simulink model "k1vissr2p"  (Simulink 8.6)
settings: Solver=ode45  StartTime=0.0  StopTime=10.0  RelTol=1e-3
libraries: cdsIPCx x11, cdsCDI64 x3, cdsCDO64 x3, TYPEB_MASTER x3, dac x2, cdsAdcx0 x1, cdsParameters x1
settings Model: Creator=controls  LastModifiedBy=controls
settings DataIOCC: SignalLoggingSaveFormat=Dataset
settings OptimizationCC: ExpressionDepthLimit=128
settings DebuggingCC: UnderspecifiedInitializationDetection=Simplified  MergeDetectMultiDrivingBlocksExec=error  SolverPrmCheckMsg=none  FcnCallInpInsideContextMsg=EnableAllAsError  StateNameClashWarn=none
settings GRTTargetCC: CombineOutputUpdateFcns=on  GRTInterface=off

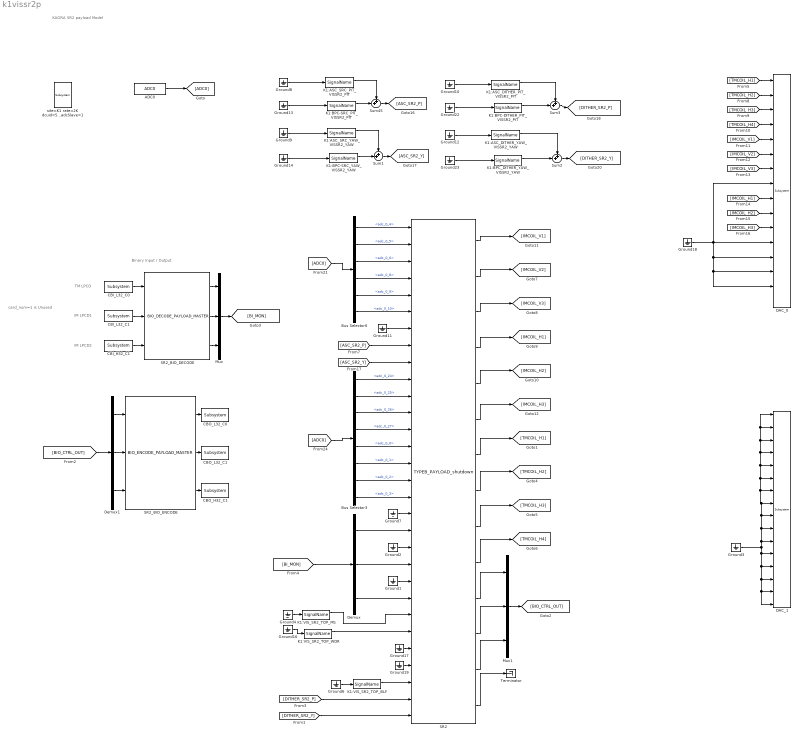
== system k1vissr2p ==
  note: KAGRA SR2 payload Model
  note: TM LPCD
  note: Binary Input / Output
  note: card_num=1 is Unused
  note: IM LPCD1
  note: IM LPCD2
  ADC0 : cdsAdcx0/ADC0  Tag=cdsAdc  Description=|
      | type-GSC_16AI64SSA
      | card_num=0
      settings: AttributesFormatString=%<Description>\n%<Tag>
  Bus Selector3 : BusSelector  Description=ADC Selector  OutputSignals=adc_0_24,adc_0_25,adc_0_26,adc_0_27,adc_0_0,adc_0_1,adc_0_2,adc_0_3
      settings: AttributesFormatString=%<Description>
  Bus Selector6 : BusSelector  Description=ADC Selector  OutputSignals=adc_0_4,adc_0_5,adc_0_6,adc_0_8,adc_0_9,adc_0_10
      settings: AttributesFormatString=%<Description>
  CBI_H32_C1 : cdsCDI64/Subsystem  Tag=cdsCDI64  Description=card_num=3
      settings: AttributesFormatString=%<Tag>\n%<Description>
  CBI_L32_C0 : cdsCDI64/Subsystem  Tag=cdsCDI64  Description=card_num=0
      settings: AttributesFormatString=%<Tag>\n%<Description>
  CBI_L32_C1 : cdsCDI64/Subsystem  Tag=cdsCDI64  Description=card_num=2
      settings: AttributesFormatString=%<Tag>\n%<Description>
  CBO_H32_C1 : cdsCDO64/Subsystem  Tag=cdsCDO64  Description=card_num=3
      settings: AttributesFormatString=%<Tag>\n%<Description>
  CBO_L32_C0 : cdsCDO64/Subsystem  Tag=cdsCDO64  Description=card_num=0
      settings: AttributesFormatString=%<Tag>\n%<Description>
  CBO_L32_C1 : cdsCDO64/Subsystem  Tag=cdsCDO64  Description=card_num=2
      settings: AttributesFormatString=%<Tag>\n%<Description>
  DAC_0 : dac/Subsystem  Description=|
      | type=GSC_16AO16,
      | card_num=0
      settings: AttributesFormatString=%<Description>
  DAC_1 : dac/Subsystem  Description=|
      | type=GSC_16AO16,
      | card_num=1
      settings: AttributesFormatString=%<Description>
  Demux : Demux  Outputs=3
  Demux1 : Demux  Outputs=3
  Ground{1..4,6..14,16..19,22..23} (19 alike) : Ground
  K1:ASC_DITHER_PIT_VISSR2_PIT : cdsIPCx/SignalName  Tag=cdsIPCx_PCIE  Description=Inter-Process Communication via PCI Express network.
      settings: AttributesFormatString=%<Tag>
  K1:ASC_DITHER_YAW_VISSR2_YAW : cdsIPCx/SignalName  Tag=cdsIPCx_PCIE  Description=Inter-Process Communication via PCI Express network.
      settings: AttributesFormatString=%<Tag>
  K1:ASC_SRC_PIT_VISSR2_PIT : cdsIPCx/SignalName  Tag=cdsIPCx_PCIE  Description=Inter-Process Communication via PCI Express network.
      settings: AttributesFormatString=%<Tag>
  K1:ASC_SRC_YAW_VISSR2_YAW : cdsIPCx/SignalName  Tag=cdsIPCx_PCIE  Description=Inter-Process Communication via PCI Express network.
      settings: AttributesFormatString=%<Tag>
  K1:BPC-DITHER_PIT_VISSR2_PIT : cdsIPCx/SignalName  Tag=cdsIPCx_PCIE  Description=Inter-Process Communication via PCI Express network.
      settings: AttributesFormatString=%<Tag>
  K1:BPC-SRC_PIT_VISSR2_PIT : cdsIPCx/SignalName  Tag=cdsIPCx_PCIE  Description=Inter-Process Communication via PCI Express network.
      settings: AttributesFormatString=%<Tag>
  K1:BPC-SRC_YAW_VISSR2_YAW : cdsIPCx/SignalName  Tag=cdsIPCx_PCIE  Description=Inter-Process Communication via PCI Express network.
      settings: AttributesFormatString=%<Tag>
  K1:BPC_DITHER_YAW_VISSR2_YAW : cdsIPCx/SignalName  Tag=cdsIPCx_PCIE  Description=Inter-Process Communication via PCI Express network.
      settings: AttributesFormatString=%<Tag>
  K1:VIS_SR2_TOP_BLF : cdsIPCx/SignalName  Tag=cdsIPCx_SHMEM  Description=Inter-Process Communication via Shared memory.
      settings: AttributesFormatString=%<Tag>
  K1:VIS_SR2_TOP_MS : cdsIPCx/SignalName  Tag=cdsIPCx_SHMEM  Description=Inter-Process Communication via Shared memory.
      settings: AttributesFormatString=%<Tag>
  K1:VIS_SR2_TOP_WDR : cdsIPCx/SignalName  Tag=cdsIPCx_SHMEM  Description=Inter-Process Communication via Shared memory.
      settings: AttributesFormatString=%<Tag>
  Mux : Mux  Inputs=3
  Mux1 : Mux  Inputs=3
  SR2 : TYPEB_MASTER/TYPEB_PAYLOAD_shutdown
  SR2_BIO_DECODE : TYPEB_MASTER/BIO_DECODE_PAYLOAD_MASTER
  SR2_BIO_ENCODE : TYPEB_MASTER/BIO_ENCODE_PAYLOAD_MASTER
  Sum{1..3,45} (4 alike) : Sum  Inputs=++|
  Terminator : Terminator
  site=K1 rate=2K dcuid=55 host=k1sr2 specific_cpu=5 adcSlave=1 : cdsParameters/Subsystem  Tag=cdsParameters  Description=|
      | Purpose:                                                                                                                                                                                                                                
      | Provide system parameters to the FE code generator to properly configure the generated EPICS names, rep rate of the FE controller, and the Data Acquisition node ID for proper storage of data from this FE controller.                 
      |                                                                                                                                                                                                                                         
      | Useage:                                                                                                                                                                                                                                 
      | The part NAME field is used to identify the FE parameters. It must be of the form:                                                                                                                                                      
      | site=                                                                                                                                                                                                                                   
      | rate=                                                                                                                                                                                                                                   
      | dcuid=                                                                                                                                                                                                                                  
      |                                                                                                                                                                                                                                         
      | Where:                                                                                                                                                                                                                                  
      | site= argument may be H1, H2, L1, M1, G1, either as a single argument or multiple, for example site=H1,H2. These are the only names allowed. These will become the first two characters of all EPICS and signal names (for example G1:).
      |                                                                                                                                                                                                                                         
      | rate= may be 2K, 16K, 32K, or 64K                                                                                                                                                                                                       
      |                                                                                                                                                                                                                                         
      | dcuid= is site specific ie it must be unique at each site.
      settings: AttributesFormatString=%<Tag>
  wires:
  ADC0/1 -> [ADC0]
  [ADC0] -> Bus Selector6/1
  SR2/10 -> [TMCOIL_H4]
  SR2/9 -> [TMCOIL_H3]
  SR2/8 -> [TMCOIL_H2]
  SR2/7 -> [TMCOIL_H1]
  SR2/1 -> [IMCOIL_V1]
  SR2/2 -> [IMCOIL_V2]
  SR2/3 -> [IMCOIL_V3]
  SR2/4 -> [IMCOIL_H1]
  SR2/5 -> [IMCOIL_H2]
  SR2/6 -> [IMCOIL_H3]
  Ground18/1 -> DAC_0/12, DAC_0/13, DAC_0/14, DAC_0/15, DAC_0/8
  Bus Selector6/1 -> SR2/1  "<adc_0_4>"
  Bus Selector6/2 -> SR2/2  "<adc_0_5>"
  Bus Selector6/3 -> SR2/3  "<adc_0_6>"
  [TMCOIL_H2] -> DAC_0/2
  [TMCOIL_H3] -> DAC_0/3
  [TMCOIL_H1] -> DAC_0/1
  [TMCOIL_H4] -> DAC_0/4
  [IMCOIL_V1] -> DAC_0/5
  [IMCOIL_V2] -> DAC_0/6
  [IMCOIL_V3] -> DAC_0/7
  Bus Selector6/4 -> SR2/4  "<adc_0_8>"
  Bus Selector6/5 -> SR2/5  "<adc_0_9>"
  Bus Selector6/6 -> SR2/6  "<adc_0_10>"
  [IMCOIL_H3] -> DAC_0/11
  [IMCOIL_H2] -> DAC_0/10
  [IMCOIL_H1] -> DAC_0/9
  [ADC0] -> Bus Selector3/1
  Bus Selector3/1 -> SR2/10  "<adc_0_24>"
  Bus Selector3/2 -> SR2/11  "<adc_0_25>"
  Bus Selector3/3 -> SR2/12  "<adc_0_26>"
  Bus Selector3/4 -> SR2/13  "<adc_0_27>"
  SR2_BIO_ENCODE/1 -> CBO_L32_C0/1
  SR2_BIO_ENCODE/3 -> CBO_H32_C1/1
  SR2_BIO_ENCODE/2 -> CBO_L32_C1/1
  CBI_L32_C1/1 -> SR2_BIO_DECODE/2
  CBI_H32_C1/1 -> SR2_BIO_DECODE/3
  SR2_BIO_DECODE/2 -> Mux/2
  SR2_BIO_DECODE/3 -> Mux/3
  SR2_BIO_DECODE/1 -> Mux/1
  Mux/1 -> [BI_MON]
  Demux1/2 -> SR2_BIO_ENCODE/2
  Demux1/3 -> SR2_BIO_ENCODE/3
  Demux1/1 -> SR2_BIO_ENCODE/1
  [BIO_CTRL_OUT] -> Demux1/1
  Mux1/1 -> [BIO_CTRL_OUT]
  [BI_MON] -> Demux/1
  Demux/1 -> SR2/19
  Demux/2 -> SR2/21
  Demux/3 -> SR2/23
  Ground7/1 -> SR2/18
  Ground1/1 -> SR2/22
  Ground2/1 -> SR2/20
  Ground3/1 -> DAC_1/13, DAC_1/14, DAC_1/15, DAC_1/16, DAC_1/12, DAC_1/7, DAC_1/6, DAC_1/5, DAC_1/1, DAC_1/2, DAC_1/3, DAC_1/4, DAC_1/8, DAC_1/9, DAC_1/10, DAC_1/11
  Bus Selector3/5 -> SR2/14  "<adc_0_0>"
  Bus Selector3/6 -> SR2/15  "<adc_0_1>"
  Bus Selector3/7 -> SR2/16  "<adc_0_2>"
  Bus Selector3/8 -> SR2/17  "<adc_0_3>"
  Ground17/1 -> SR2/26
  Ground19/1 -> SR2/27
  CBI_L32_C0/1 -> SR2_BIO_DECODE/1
  Ground6/1 -> K1:VIS_SR2_TOP_BLF/1
  K1:VIS_SR2_TOP_BLF/1 -> SR2/28
  SR2/13 -> Mux1/3
  SR2/12 -> Mux1/2
  SR2/11 -> Mux1/1
  SR2/14 -> Terminator/1
  Ground11/1 -> SR2/7
  [ASC_SR2_P] -> SR2/8
  [DITHER_SR2_P] -> SR2/29
  [DITHER_SR2_Y] -> SR2/30
  Sum45/1 -> [ASC_SR2_P]
  K1:ASC_SRC_PIT_VISSR2_PIT/1 -> Sum45/1
  Sum1/1 -> [ASC_SR2_Y]
  K1:ASC_SRC_YAW_VISSR2_YAW/1 -> Sum1/1
  K1:BPC-SRC_YAW_VISSR2_YAW/1 -> Sum1/2
  K1:BPC-SRC_PIT_VISSR2_PIT/1 -> Sum45/2
  Sum3/1 -> [DITHER_SR2_P]
  K1:ASC_DITHER_PIT_VISSR2_PIT/1 -> Sum3/1
  Sum2/1 -> [DITHER_SR2_Y]
  K1:ASC_DITHER_YAW_VISSR2_YAW/1 -> Sum2/1
  K1:BPC-DITHER_PIT_VISSR2_PIT/1 -> Sum3/2
  Ground22/1 -> K1:BPC-DITHER_PIT_VISSR2_PIT/1
  Ground23/1 -> K1:BPC_DITHER_YAW_VISSR2_YAW/1
  K1:BPC_DITHER_YAW_VISSR2_YAW/1 -> Sum2/2
  Ground8/1 -> K1:ASC_SRC_PIT_VISSR2_PIT/1
  Ground9/1 -> K1:ASC_SRC_YAW_VISSR2_YAW/1
  Ground10/1 -> K1:ASC_DITHER_PIT_VISSR2_PIT/1
  Ground12/1 -> K1:ASC_DITHER_YAW_VISSR2_YAW/1
  Ground13/1 -> K1:BPC-SRC_PIT_VISSR2_PIT/1
  Ground14/1 -> K1:BPC-SRC_YAW_VISSR2_YAW/1
  [ASC_SR2_Y] -> SR2/9
  Ground16/1 -> K1:VIS_SR2_TOP_WDR/1
  Ground4/1 -> K1:VIS_SR2_TOP_MS/1
  K1:VIS_SR2_TOP_MS/1 -> SR2/24
  K1:VIS_SR2_TOP_WDR/1 -> SR2/25
